simulink model "Feedback_Configuration_1"  (R2020b)
settings: Solver=VariableStepAuto  StartTime=0.0  StopTime=10.0  RelTol=1e-3
libraries: cstblocks x4
settings Model: Creator=danielcastro  LastModifiedBy=danielcastro

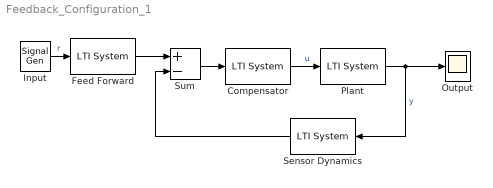
== system Feedback_Configuration_1 ==
  Compensator : cstblocks/LTI System  sys=C  IC=[]
  Feed Forward : cstblocks/LTI System  sys=F  IC=[]
  Input : SignalGenerator
  Output : Scope
  Plant : cstblocks/LTI System  sys=G  IC=[]
  Sensor Dynamics : cstblocks/LTI System  sys=H  IC=[]
  Sum : Sum  Inputs=+-
  wires:
  Input/1 -> Feed Forward/1  "r"
  Feed Forward/1 -> Sum/1
  Sensor Dynamics/1 -> Sum/2
  Sum/1 -> Compensator/1
  Compensator/1 -> Plant/1  "u"
  Plant/1 -> Output/1, Sensor Dynamics/1  "y"
